simulink model "dycos10_induction_1"  (Simulink 9.2)
settings: Solver=VariableStepAuto  StartTime=0.0  StopTime=19  RelTol=1e-3
undefined symbols (not defined in the file): D1, Delta, k1, k2
libraries: powerlib x49, powerlib_meascontrol x2, factslib x1
settings Model: Creator=moham  LastModifiedBy=moham
settings DataIOCC: LimitDataPoints=off  SaveFormat=Dataset  SignalLoggingSaveFormat=Dataset  ReturnWorkspaceOutputs=on
settings OptimizationCC: LifeSpan=auto
settings DebuggingCC: UnderspecifiedInitializationDetection=Simplified  MergeDetectMultiDrivingBlocksExec=error  FcnCallInpInsideContextMsg=error  UnconnectedInputMsg=none  UnconnectedOutputMsg=none  UnconnectedLineMsg=none  StateNameClashWarn=none  SFUnexpectedBacktrackingDiag=error  SFNoUnconditionalDefaultTransitionDiag=error  SFExecutionAtInitializationDiag=warning
settings HardwareCC: ProdBitPerPointer=64  ProdBitPerSizeT=64  ProdBitPerPtrDiffT=64  ProdLargestAtomicFloat=Float  ProdIntDivRoundTo=Zero  ProdEndianess=LittleEndian  ProdWordSize=64  ProdHWDeviceType=Intel->x86-64 (Windows64)
settings ModelReferenceCC: EnableRefExpFcnMdlSchedulingChecks=off  PropagateSignalLabelsOutOfModel=on
settings SFSimCC: SimUseLocalCustomCode=on
settings RTWCC: RTWUseLocalCustomCode=on
settings CodeAppCC: StateflowObjectComments=off
settings GRTTargetCC: TargetLangStandard=C99 (ISO)  CombineOutputUpdateFcns=on  GRTInterface=off
settings ConfigComp: CovMetricSettings=dwe  CovSaveCumulativeToWorkspaceVar=off  CovSaveSingleToWorkspaceVar=off  CovExternalEMLEnable=on

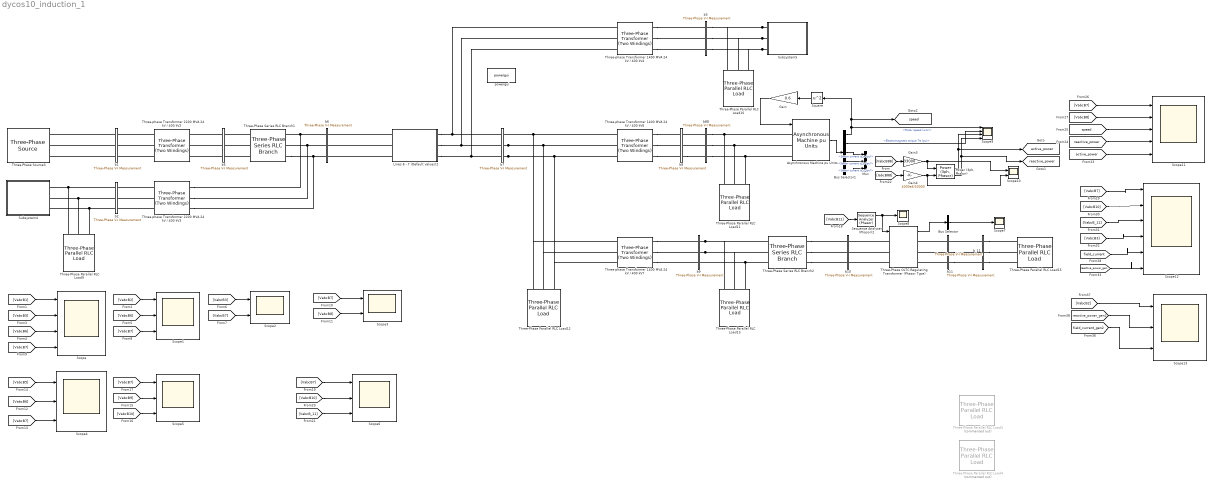
== system dycos10_induction_1 ==
  Asynchronous Machine pu Units : powerlib/Machines/Asynchronous Machine pu Units  RotorType=Squirrel-cage  PresetModel=No  MechanicalLoad=Torque Tm  ShowDetailedParameters=on  ReferenceFrame=Rotor  Units=pu  MeasurementBus=off  NominalParameters=[3600e6 33000 60]  VoltageRatio=1  Stator=[0.01 0.145]  Rotor=[0.008 0.145]  Cage1=[0.01909 0.0397]  Cage2=[0.01909 0.0397]  Lm=3.3  Mechanical=[0.6 0 2]  PolePairs=2  InitialConditions=[-6.39894e-41 0 0.310738 0.310738 0.310738 -24.5903 -144.59 95.4097]  SimulateSaturation=off  Saturation="[0.212,0.4201,0.8125,1.0979,1.4799,2.2457,3.2586,4.5763,6.4763 ;   0.5,0.7,0.9,1,1.1,1.2 ,1.3,1.4,1.5]"  LoadFlowParameters=0  TsPowergui=0  TsBlock=-1  IterativeModel=Trapezoidal non iterative  IterativeDiscreteModel=Trapezoidal non iterative  Pmec=3600e6*0.6
  Bus Selector : BusSelector  OutputSignals=Tap  OutputAsBus=on
  Bus Selector1 : BusSelector  OutputSignals=Mechanical.Rotor speed (wm),Mechanical.Electromagnetic torque Te (pu),Stator measurements.Stator current is_a (pu),Stator measurements.Stator current is_b (pu),Stator measurements.Stator current is_c (pu)
  Gain : Gain  Gain=0.6
  Gain3 : Gain  Gain=33000
  Gain4 : Gain  Gain=4000e6/33000
  Lines 6 - 7 (Default values)2 : Subsystem
  Mux : Mux  Inputs=3
  "Power (3ph, Phasor)" : powerlib_meascontrol/Measurements/Power (3ph, Phasor)
  Scope : Scope  NumInputPorts=4
  Scope{1,4..6,13} (5 alike) : Scope  NumInputPorts=3
  Scope10 : Scope  NumInputPorts=2
  Scope11 : Scope  NumInputPorts=5
  Scope12 : Scope  NumInputPorts=6
  Scope2 : Scope  NumInputPorts=2
  Scope3 : Scope  NumInputPorts=2
  Scope7 : Scope
  Scope8 : Scope
  Scope9 : Scope  NumInputPorts=4
  Sequence Analyzer (Phasor)2 : powerlib_meascontrol/Measurements/Sequence Analyzer (Phasor)  seq=Positive
  Square : Math  Operator=square  SaturateOnIntegerOverflow=on
  Subsystem4 : Subsystem
  Subsystem5 : Subsystem
  Three-Phase Parallel RLC Load10 : powerlib/Elements/Three-Phase Parallel RLC Load  LConnTagsString=A|B|C  Configuration=Y (grounded)  NominalVoltage=(24000)*1  Vabc=[1e3 1e3 1e3]  Vabcp=[1e3 1e3 1e3]  NominalFrequency=60  UnbalancedPower=off  ActivePower=5e6  InductivePower=0  CapacitivePower=0  Pabc=[10e3 9e3 11e3]  QLabc=[100 90 110]  QCabc=[100 90 110]  Pabcp=[10e3 9e3 11e3]  QLabcp=[100 90 110]  QCabcp=[100 90 110]  Measurements=None  LoadType=constant PQ
  Three-Phase Parallel RLC Load11 : powerlib/Elements/Three-Phase Parallel RLC Load  LConnTagsString=A|B|C  Configuration=Y (grounded)  NominalVoltage=(717697)*0.0445324  Vabc=[1e3 1e3 1e3]  Vabcp=[1e3 1e3 1e3]  NominalFrequency=60  UnbalancedPower=off  ActivePower=0  InductivePower=0  CapacitivePower=600*1e6  Pabc=[10e3 9e3 11e3]  QLabc=[100 90 110]  QCabc=[100 90 110]  Pabcp=[10e3 9e3 11e3]  QLabcp=[100 90 110]  QCabcp=[100 90 110]  Measurements=None  LoadType=constant PQ
  Three-Phase Parallel RLC Load12 : powerlib/Elements/Three-Phase Parallel RLC Load  LConnTagsString=A|B|C  Configuration=Y (grounded)  NominalVoltage=(8.15772e+06)*0.0445322  Vabc=[1e3 1e3 1e3]  Vabcp=[1e3 1e3 1e3]  NominalFrequency=60  UnbalancedPower=off  ActivePower=0  InductivePower=0  CapacitivePower=763*1e6  Pabc=[10e3 9e3 11e3]  QLabc=[100 90 110]  QCabc=[100 90 110]  Pabcp=[10e3 9e3 11e3]  QLabcp=[100 90 110]  QCabcp=[100 90 110]  Measurements=None  LoadType=constant PQ
  Three-Phase Parallel RLC Load13 : powerlib/Elements/Three-Phase Parallel RLC Load  LConnTagsString=A|B|C  Configuration=Y (grounded)  NominalVoltage=(726764)*0.0445322  Vabc=[1e3 1e3 1e3]  Vabcp=[1e3 1e3 1e3]  NominalFrequency=60  UnbalancedPower=off  ActivePower=0  InductivePower=0  CapacitivePower=1710*1e6  Pabc=[10e3 9e3 11e3]  QLabc=[100 90 110]  QCabc=[100 90 110]  Pabcp=[10e3 9e3 11e3]  QLabcp=[100 90 110]  QCabcp=[100 90 110]  Measurements=None  LoadType=constant PQ
  Three-Phase Parallel RLC Load15 : powerlib/Elements/Three-Phase Parallel RLC Load  LConnTagsString=A|B|C  Configuration=Y (grounded)  NominalVoltage=11e3  Vabc=[1e3 1e3 1e3]  Vabcp=[1e3 1e3 1e3]  NominalFrequency=60  UnbalancedPower=off  ActivePower=3435*1e6  InductivePower=985*1e6  CapacitivePower=0  Pabc=[10e3 9e3 11e3]  QLabc=[100 90 110]  QCabc=[100 90 110]  Pabcp=[10e3 9e3 11e3]  QLabcp=[100 90 110]  QCabcp=[100 90 110]  Measurements=None  LoadType=constant PQ
  Three-Phase Parallel RLC Load3 : powerlib/Elements/Three-Phase Parallel RLC Load  Commented=on  LConnTagsString=A|B|C  Configuration=Y (grounded)  NominalVoltage=11e3  Vabc=[1e3 1e3 1e3]  Vabcp=[1e3 1e3 1e3]  NominalFrequency=60  UnbalancedPower=off  ActivePower=k1*0.5*1e6  InductivePower=k2*0.5*1e6  CapacitivePower=0  Pabc=[10e3 9e3 11e3]  QLabc=[100 90 110]  QCabc=[100 90 110]  Pabcp=[10e3 9e3 11e3]  QLabcp=[100 90 110]  QCabcp=[100 90 110]  Measurements=None  LoadType=constant Z
  Three-Phase Parallel RLC Load4 : powerlib/Elements/Three-Phase Parallel RLC Load  Commented=on  LConnTagsString=A|B|C  Configuration=Y (grounded)  NominalVoltage=11e3  Vabc=[1e3 1e3 1e3]  Vabcp=[1e3 1e3 1e3]  NominalFrequency=60  UnbalancedPower=off  ActivePower=k1*0.5*1e6  InductivePower=k2*0.5*1e6  CapacitivePower=0  Pabc=[10e3 9e3 11e3]  QLabc=[100 90 110]  QCabc=[100 90 110]  Pabcp=[10e3 9e3 11e3]  QLabcp=[100 90 110]  QCabcp=[100 90 110]  Measurements=None  LoadType=constant I
  Three-Phase Parallel RLC Load9 : powerlib/Elements/Three-Phase Parallel RLC Load  LConnTagsString=A|B|C  Configuration=Y (grounded)  NominalVoltage=(24000)*1  Vabc=[1e3 1e3 1e3]  Vabcp=[1e3 1e3 1e3]  NominalFrequency=60  UnbalancedPower=off  ActivePower=5e6  InductivePower=0  CapacitivePower=0  Pabc=[10e3 9e3 11e3]  QLabc=[100 90 110]  QCabc=[100 90 110]  Pabcp=[10e3 9e3 11e3]  QLabcp=[100 90 110]  QCabcp=[100 90 110]  Measurements=None  LoadType=constant PQ
  Three-Phase Series RLC Branch1 : powerlib/Elements/Three-Phase Series RLC Branch  LConnTagsString=A|B|C  RConnTagsString=A|B|C  BranchType=L  Resistance=1  Inductance=1e-3  Capacitance=1e-6  Measurements=None
  Three-Phase Series RLC Branch2 : powerlib/Elements/Three-Phase Series RLC Branch  LConnTagsString=A|B|C  RConnTagsString=A|B|C  BranchType=RL  Resistance=0.005  Inductance=0.08e-3  Capacitance=1e-6  Measurements=None
  Three-Phase OLTC Regulating Transformer (Phasor Type) : factslib/Transformers/Three-Phase OLTC Regulating Transformer (Phasor Type)  Winding1Connection=Yg  Winding2Connection=Yg  PnomFnom="[4000e6,  60]"  Winding1=[33e3, 0 , 0.001*40 ]  Winding2="[11e3,  0, 0.001*40 ]"  Iw2_init=[0.75/528, -45]  RmXm=[500, 500]  TapOnWinding=Winding 2  WindingTap=[ 0, 0.0001*40]  dU=0.00625  TapMinMax=[ -16, +16]  InitialTap=0  TapSelectionTime=1.5  ExternalControl=off  RegulatorOn=on  Regulator="[.84,  0.01, 0]"
      link override Rm_Xm_1: ActivePower=4000000  InductivePower=4000000
      link override Rm_Xm_2: ActivePower=4000000  InductivePower=4000000
  Three-Phase Source3 : powerlib/Electrical Sources/Three-Phase Source  InternalConnection=Yg  VoltagePhases=off  Voltage=(24000)*1  PhaseAngle=0  Voltage_phases=[25e3 25e3 25e3]/sqrt(3)  PhaseAngles_phases=[0 -120 +120]  Frequency=60  NonIdealSource=off  SpecifyImpedance=off  Resistance=0.8929  Inductance=16.58e-3  ShortCircuitLevel=100e6  BaseVoltage=24e3  XRratio=7  BusType=swing  Pref=50000000000  Qref=0  Prefabc=[10e3, 10e3, 10e3]  Qrefabc=[0, 0, 0]  Qmin=-Inf  Qmax=Inf
  Three-phase Transformer 1400 MVA 24 kV / 400 kV4 : powerlib/Elements/Three-Phase Transformer (Two Windings)  Winding1Connection=Delta (D1)  Winding2Connection=Yg  CoreType=Three single-phase transformers  SetSaturation=off  Hysteresis=off  DataFile='hysteresis'  SetInitialFlux=off  Measurements=None  UNITS=pu  NominalPower=[ 1400e6 60 ]  Winding1="[ 24e3 0  0.0125*14]"  Winding2=[ 400e3*0.9024 0 0.0125*14/(17*17)]  Rm=500  Lm=500  L0=0.5  Saturation="[ 0,0  ;  0.005,1.2  ;  1.0,1.4 ]"  InitialFluxes=[ 0.8 , -0.8 , 0.7 ]  BreakLoop=off  DiscreteSolver=Trapezoidal iterative  DataType=off  TransfoNumber=0
  Three-phase Transformer 1400 MVA 24 kV / 400 kV6 : powerlib/Elements/Three-Phase Transformer (Two Windings)  Winding1Connection=Delta (D1)  Winding2Connection=Yg  CoreType=Three single-phase transformers  SetSaturation=off  Hysteresis=off  DataFile='hysteresis'  SetInitialFlux=off  Measurements=None  UNITS=pu  NominalPower=[ 4000e6 60 ]  Winding1="[ 400e3 0  0.003*40/(12*12)]"  Winding2=[ 33e3*1.0664 0 0.003*40]  Rm=500  Lm=500  L0=0.5  Saturation="[ 0,0  ;  0.005,1.2  ;  1.0,1.4 ]"  InitialFluxes=[ 0.8 , -0.8 , 0.7 ]  BreakLoop=off  DiscreteSolver=Trapezoidal iterative  DataType=off  TransfoNumber=0
  Three-phase Transformer 1400 MVA 24 kV / 400 kV7 : powerlib/Elements/Three-Phase Transformer (Two Windings)  Winding1Connection=Delta (D1)  Winding2Connection=Yg  CoreType=Three single-phase transformers  SetSaturation=off  Hysteresis=off  DataFile='hysteresis'  SetInitialFlux=off  Measurements=None  UNITS=pu  NominalPower=[ 4000e6 60 ]  Winding1="[ 400e3 0  0.0026*40/144]"  Winding2=[ 33e3*1.08 0 0.0026*40]  Rm=500  Lm=500  L0=0.5  Saturation="[ 0,0  ;  0.005,1.2  ;  1.0,1.4 ]"  InitialFluxes=[ 0.8 , -0.8 , 0.7 ]  BreakLoop=off  DiscreteSolver=Trapezoidal iterative  DataType=off  TransfoNumber=0
  Three-phase Transformer 2200 MVA 24 kV / 400 kV2 : powerlib/Elements/Three-Phase Transformer (Two Windings)  Winding1Connection=Delta (D1)  Winding2Connection=Yg  CoreType=Three single-phase transformers  SetSaturation=off  Hysteresis=off  DataFile='hysteresis'  SetInitialFlux=off  Measurements=None  UNITS=pu  NominalPower=[ 4000e6 60 ]  Winding1="[ 24e3 0  0.002/400]"  Winding2=[ 400e3*0.8857 0 0.002/400]  Rm=1000  Lm=1000  L0=0.5  Saturation="[ 0,0  ;  0.005,1.2  ;  1.0,1.4 ]"  InitialFluxes=[ 0.8 , -0.8 , 0.7 ]  BreakLoop=off  DiscreteSolver=Trapezoidal iterative  DataType=off  TransfoNumber=0
  Three-phase Transformer 2200 MVA 24 kV / 400 kV3 : powerlib/Elements/Three-Phase Transformer (Two Windings)  Winding1Connection=Delta (D1)  Winding2Connection=Yg  CoreType=Three single-phase transformers  SetSaturation=off  Hysteresis=off  DataFile='hysteresis'  SetInitialFlux=off  Measurements=None  UNITS=pu  NominalPower=[ 2200e6 60 ]  Winding1="[ 24e3 0  0.0045*22]"  Winding2=[ 400e3*0.8857 0 0.0045*22/(17*17)]  Rm=500  Lm=500  L0=0.5  Saturation="[ 0,0  ;  0.005,1.2  ;  1.0,1.4 ]"  InitialFluxes=[ 0.8 , -0.8 , 0.7 ]  BreakLoop=off  DiscreteSolver=Trapezoidal iterative  DataType=off  TransfoNumber=0
  b1 : powerlib/Measurements/Three-Phase V-I Measurement  VoltageMeasurement=phase-to-ground  SetLabelV=on  LabelV=VabcB1  Vpu=on  VpuLL=off  CurrentMeasurement=yes  SetLabelI=on  LabelI=IabcB1  Ipu=on  Pbase=4000e6  Vbase=24e3  OutputType=Magnitude  PhasorSimulation=on  PSBequivalent=0
  b10 : powerlib/Measurements/Three-Phase V-I Measurement  VoltageMeasurement=phase-to-ground  SetLabelV=on  LabelV=VabcB10  Vpu=on  VpuLL=off  CurrentMeasurement=yes  SetLabelI=on  LabelI=IabcB10  Ipu=on  Pbase=4000e6  Vbase=33e3  OutputType=Magnitude  PhasorSimulation=on  PSBequivalent=0
  b11 : powerlib/Measurements/Three-Phase V-I Measurement  VoltageMeasurement=phase-to-ground  SetLabelV=on  LabelV=VabcB11  Vpu=on  VpuLL=off  CurrentMeasurement=yes  SetLabelI=on  LabelI=IabcB11  Ipu=on  Pbase=4000e6  Vbase=11e3  OutputType=Complex  PhasorSimulation=on  PSBequivalent=0
  b2 : powerlib/Measurements/Three-Phase V-I Measurement  VoltageMeasurement=phase-to-ground  SetLabelV=on  LabelV=VabcB2  Vpu=on  VpuLL=off  CurrentMeasurement=yes  SetLabelI=on  LabelI=IabcB2  Ipu=on  Pbase=2200e6  Vbase=24e3  OutputType=Magnitude  PhasorSimulation=on  PSBequivalent=0
  b3 : powerlib/Measurements/Three-Phase V-I Measurement  VoltageMeasurement=phase-to-phase  SetLabelV=on  LabelV=VabcB3  Vpu=on  VpuLL=off  CurrentMeasurement=yes  SetLabelI=on  LabelI=IabcB3  Ipu=on  Pbase=1100e6  Vbase=24e3  OutputType=Magnitude  PhasorSimulation=on  PSBequivalent=0
  b5 : powerlib/Measurements/Three-Phase V-I Measurement  VoltageMeasurement=phase-to-ground  SetLabelV=on  LabelV=VabcB5  Vpu=on  VpuLL=off  CurrentMeasurement=yes  SetLabelI=on  LabelI=IabcB5  Ipu=on  Pbase=4000e6  Vbase=400e3  OutputType=Magnitude  PhasorSimulation=on  PSBequivalent=0
  b6 : powerlib/Measurements/Three-Phase V-I Measurement  VoltageMeasurement=phase-to-ground  SetLabelV=on  LabelV=VabcB6  Vpu=on  VpuLL=off  CurrentMeasurement=yes  SetLabelI=on  LabelI=IabcB6  Ipu=on  Pbase=4000e6  Vbase=400e3  OutputType=Magnitude  PhasorSimulation=on  PSBequivalent=0
  b7 : powerlib/Measurements/Three-Phase V-I Measurement  VoltageMeasurement=phase-to-ground  SetLabelV=on  LabelV=VabcB7  Vpu=on  VpuLL=off  CurrentMeasurement=yes  SetLabelI=on  LabelI=IabcB7  Ipu=on  Pbase=4000e6  Vbase=400e3  OutputType=Magnitude  PhasorSimulation=on  PSBequivalent=0
  b8 : powerlib/Measurements/Three-Phase V-I Measurement  VoltageMeasurement=phase-to-ground  SetLabelV=on  LabelV=VabcB8  Vpu=on  VpuLL=off  CurrentMeasurement=yes  SetLabelI=on  LabelI=IabcB8  Ipu=on  Pbase=4000e6  Vbase=33e3  OutputType=Magnitude  PhasorSimulation=on  PSBequivalent=0
  b88 : powerlib/Measurements/Three-Phase V-I Measurement  VoltageMeasurement=phase-to-ground  SetLabelV=on  LabelV=VabcB88  Vpu=on  VpuLL=off  CurrentMeasurement=yes  SetLabelI=on  LabelI=IabcB88  Ipu=on  Pbase=4000e6  Vbase=33e3  OutputType=Complex  PhasorSimulation=on  PSBequivalent=0
  b9 : powerlib/Measurements/Three-Phase V-I Measurement  VoltageMeasurement=phase-to-ground  SetLabelV=on  LabelV=VabcB9  Vpu=on  VpuLL=off  CurrentMeasurement=yes  SetLabelI=on  LabelI=IabcB9  Ipu=on  Pbase=4000e6  Vbase=33e3  OutputType=Magnitude  PhasorSimulation=on  PSBequivalent=0
  b_11 : powerlib/Measurements/Three-Phase V-I Measurement  VoltageMeasurement=phase-to-ground  SetLabelV=on  LabelV=VabcB_11  Vpu=on  VpuLL=off  CurrentMeasurement=yes  SetLabelI=on  LabelI=IabcB_11  Ipu=on  Pbase=4000e6  Vbase=11e3  OutputType=Magnitude  PhasorSimulation=on  PSBequivalent=0
  powergui : powerlib/powergui  Priority=1  SimulationMode=Phasor  SampleTime=5e-6  frequency=60  Iterations=50  frequencyindice=60  Pbase=100e6  ErrMax=1e-4  UnitsV=kV  UnitsW=MW  buscounter=0  FunctionMessages=off  echomessages=off  EnableUseOfTLC=off  CurrentSourceSwitches=off  DisableSnubberDevices=off  DisableRonSwitches=off  DisableVfSwitches=off  DisplayEquations=off  AutomaticDiscreteSolvers=off  SolverType=Tustin/Backward Euler (TBE)  Interpol=off  ExternalGateDelay=off  methode=off  Ts=100  x0status=blocks  SPID=on  SwTol=0  HookPort=off  NonlinearTolerance=1e-4  nMaxIteration=100  ContinueOnMaxIteration=off  RestoreLinks=warning  ResistiveCurrentMeasurement=off  Frange=[0:2:500]  Ylog=off  Xlog=on  ShowGrid=off  save=off  variable=ZData  structure=0  ZoomFFT=off  StartTime=0.0  cycles=1  DisplayStyle=1  fundamental=60  FreqAxis=off  MaxFrequency=1000  frequencyindicesteady=1  RmsSteady=1  display=off
  tag scope: active_power=global, reactive_power=global, speed=global
  wires:
  [VabcB7] -> Scope6/1
  [VabcB10] -> Scope6/2
  [VabcB7] -> Scope/4
  Bus Selector/1 -> Scope7/1
  Sequence Analyzer (Phasor)2/1 -> Scope8/1, Three-Phase OLTC Regulating Transformer (Phasor Type)/1
  [VabcB7] -> Scope5/1
  [VabcB11] -> Sequence Analyzer (Phasor)2/1
  [VabcB7] -> Scope2/2
  [VabcB2] -> Scope1/1
  [VabcB10] -> Scope5/3
  [VabcB3] -> Scope2/1
  [VabcB5] -> Scope4/1
  [VabcB9] -> Scope5/2
  [VabcB5] -> Scope/2
  [VabcB7] -> Scope4/3
  Three-Phase OLTC Regulating Transformer (Phasor Type)/1 -> Bus Selector/1
  [VabcB6] -> Scope4/2
  [VabcB7] -> Scope3/1
  [VabcB7] -> Scope1/3
  [VabcB_11] -> Scope6/3
  [VabcB1] -> Scope/1
  [VabcB6] -> Scope1/2
  [VabcB8] -> Scope3/2
  [VabcB6] -> Scope/3
  Asynchronous Machine pu Units/1 -> Bus Selector1/1
  Bus Selector1/1 -> [speed], Square/1, Scope9/1  "<Rotor speed (wm)>"
  Square/1 -> Gain/1
  Gain/1 -> Asynchronous Machine pu Units/1
  Bus Selector1/2 -> Scope9/2  "<Electromagnetic torque Te (pu)>"
  Bus Selector1/3 -> Mux/1  "<Stator current is_a (pu)>"
  Bus Selector1/4 -> Mux/2  "<Stator current is_b (pu)>"
  Bus Selector1/5 -> Mux/3  "<Stator current is_c (pu)>"
  "Power (3ph, Phasor)"/1 -> [active_power], Scope9/3
  "Power (3ph, Phasor)"/2 -> [reactive_power], Scope9/4
  Gain4/1 -> "Power (3ph, Phasor)"/2, Scope10/2
  Gain3/1 -> "Power (3ph, Phasor)"/1, Scope10/1
  [VabcB88] -> Gain3/1
  [IabcB88] -> Gain4/1
  [VabcB7] -> Scope11/1
  [VabcB8] -> Scope11/2
  [speed] -> Scope11/3
  [reactive_power] -> Scope11/4
  [active_power] -> Scope11/5
  [VabcB_11] -> Scope12/3
  [field_current] -> Scope12/5
  [VabcB10] -> Scope12/2
  [VabcB7] -> Scope12/1
  [VabcB3] -> Scope12/4
  [reactive_power_gen] -> Scope12/6
  [field_current_gen2] -> Scope13/3
  [reactive_power_gen2] -> Scope13/2
  [VabcB2] -> Scope13/1
  connections:
  Three-phase Transformer 1400 MVA 24 kV / 400 kV6/LConn1 -- Three-Phase Parallel RLC Load12/LConn1 -- Three-phase Transformer 1400 MVA 24 kV / 400 kV7/LConn1 -- b7/RConn1
  Three-phase Transformer 2200 MVA 24 kV / 400 kV3/RConn1 -- b6/LConn1 -- Three-Phase Series RLC Branch1/RConn1
  Subsystem5/RConn2 -- Three-Phase Parallel RLC Load10/LConn2 -- b3/LConn2
  Three-Phase Parallel RLC Load13/LConn3 -- b9/RConn3 -- Three-Phase Series RLC Branch2/LConn3
  Three-phase Transformer 2200 MVA 24 kV / 400 kV3/RConn2 -- b6/LConn2 -- Three-Phase Series RLC Branch1/RConn2
  b7/RConn2 -- Three-Phase Parallel RLC Load12/LConn2 -- Three-phase Transformer 1400 MVA 24 kV / 400 kV7/LConn2 -- Three-phase Transformer 1400 MVA 24 kV / 400 kV6/LConn2
  Lines 6 - 7 (Default values)2/RConn2 -- Three-phase Transformer 1400 MVA 24 kV / 400 kV4/RConn2 -- b7/LConn2
  Three-Phase Series RLC Branch1/RConn3 -- Three-phase Transformer 2200 MVA 24 kV / 400 kV3/RConn3 -- b6/LConn3
  b7/RConn3 -- Three-Phase Parallel RLC Load12/LConn3 -- Three-phase Transformer 1400 MVA 24 kV / 400 kV7/LConn3 -- Three-phase Transformer 1400 MVA 24 kV / 400 kV6/LConn3
  b9/RConn1 -- Three-Phase Parallel RLC Load13/LConn1 -- Three-Phase Series RLC Branch2/LConn1
  Three-Phase Parallel RLC Load9/LConn3 -- b2/LConn3 -- Subsystem4/RConn3
  Three-Phase Parallel RLC Load9/LConn1 -- b2/LConn1 -- Subsystem4/RConn1
  Lines 6 - 7 (Default values)2/RConn1 -- Three-phase Transformer 1400 MVA 24 kV / 400 kV4/RConn1 -- b7/LConn1
  Subsystem5/RConn3 -- b3/LConn3 -- Three-Phase Parallel RLC Load10/LConn3
  Subsystem5/RConn1 -- Three-Phase Parallel RLC Load10/LConn1 -- b3/LConn1
  Three-Phase Parallel RLC Load9/LConn2 -- b2/LConn2 -- Subsystem4/RConn2
  b88/LConn2 -- b8/RConn2
  b88/LConn1 -- b8/RConn1
  Lines 6 - 7 (Default values)2/RConn3 -- Three-phase Transformer 1400 MVA 24 kV / 400 kV4/RConn3 -- b7/LConn3
  b9/RConn2 -- Three-Phase Parallel RLC Load13/LConn2 -- Three-Phase Series RLC Branch2/LConn2
  Three-Phase Parallel RLC Load11/LConn3 -- Asynchronous Machine pu Units/LConn3 -- b88/RConn3
  Three-phase Transformer 1400 MVA 24 kV / 400 kV4/LConn1 -- b3/RConn1
  b11/RConn3 -- b_11/LConn3
  Three-phase Transformer 2200 MVA 24 kV / 400 kV2/LConn3 -- b1/RConn3
  b_11/RConn1 -- Three-Phase Parallel RLC Load15/LConn1
  b_11/RConn3 -- Three-Phase Parallel RLC Load15/LConn3
  Three-Phase Series RLC Branch2/RConn3 -- b10/LConn3
  b5/LConn3 -- Three-phase Transformer 2200 MVA 24 kV / 400 kV2/RConn3
  Three-Phase OLTC Regulating Transformer (Phasor Type)/LConn3 -- b10/RConn3
  Three-phase Transformer 1400 MVA 24 kV / 400 kV7/RConn2 -- b9/LConn2
  Three-Phase OLTC Regulating Transformer (Phasor Type)/LConn2 -- b10/RConn2
  Three-phase Transformer 1400 MVA 24 kV / 400 kV6/RConn3 -- b8/LConn3
  Three-Phase Series RLC Branch1/LConn2 -- b5/RConn2
  Three-Phase Series RLC Branch2/RConn2 -- b10/LConn2
  Three-phase Transformer 1400 MVA 24 kV / 400 kV4/LConn3 -- b3/RConn3
  Three-phase Transformer 1400 MVA 24 kV / 400 kV4/LConn2 -- b3/RConn2
  Three-Phase Series RLC Branch1/LConn1 -- b5/RConn1
  b5/LConn1 -- Three-phase Transformer 2200 MVA 24 kV / 400 kV2/RConn1
  Lines 6 - 7 (Default values)2/LConn2 -- b6/RConn2
  b_11/LConn1 -- b11/RConn1
  Three-phase Transformer 2200 MVA 24 kV / 400 kV3/LConn1 -- b2/RConn1
  Three-Phase Series RLC Branch2/RConn1 -- b10/LConn1
  Three-phase Transformer 2200 MVA 24 kV / 400 kV2/LConn1 -- b1/RConn1
  b1/LConn1 -- Three-Phase Source3/RConn1
  Lines 6 - 7 (Default values)2/LConn3 -- b6/RConn3
  b11/LConn2 -- Three-Phase OLTC Regulating Transformer (Phasor Type)/RConn2
  b11/LConn3 -- Three-Phase OLTC Regulating Transformer (Phasor Type)/RConn3
  Three-phase Transformer 1400 MVA 24 kV / 400 kV6/RConn1 -- b8/LConn1
  Three-Phase OLTC Regulating Transformer (Phasor Type)/LConn1 -- b10/RConn1
  b_11/RConn2 -- Three-Phase Parallel RLC Load15/LConn2
  Three-Phase Series RLC Branch1/LConn3 -- b5/RConn3
  b1/LConn2 -- Three-Phase Source3/RConn2
  Three-phase Transformer 2200 MVA 24 kV / 400 kV3/LConn2 -- b2/RConn2
  Three-phase Transformer 1400 MVA 24 kV / 400 kV6/RConn2 -- b8/LConn2
  Three-phase Transformer 2200 MVA 24 kV / 400 kV2/LConn2 -- b1/RConn2
  Three-phase Transformer 1400 MVA 24 kV / 400 kV7/RConn1 -- b9/LConn1
  b11/RConn2 -- b_11/LConn2
  b11/LConn1 -- Three-Phase OLTC Regulating Transformer (Phasor Type)/RConn1
  b1/LConn3 -- Three-Phase Source3/RConn3
  Three-phase Transformer 2200 MVA 24 kV / 400 kV3/LConn3 -- b2/RConn3
  Lines 6 - 7 (Default values)2/LConn1 -- b6/RConn1
  Three-phase Transformer 1400 MVA 24 kV / 400 kV7/RConn3 -- b9/LConn3
  b5/LConn2 -- Three-phase Transformer 2200 MVA 24 kV / 400 kV2/RConn2
  Three-Phase Parallel RLC Load11/LConn1 -- Asynchronous Machine pu Units/LConn1 -- b88/RConn1
  Three-Phase Parallel RLC Load11/LConn2 -- b88/RConn2 -- Asynchronous Machine pu Units/LConn2
  b8/RConn3 -- b88/LConn3

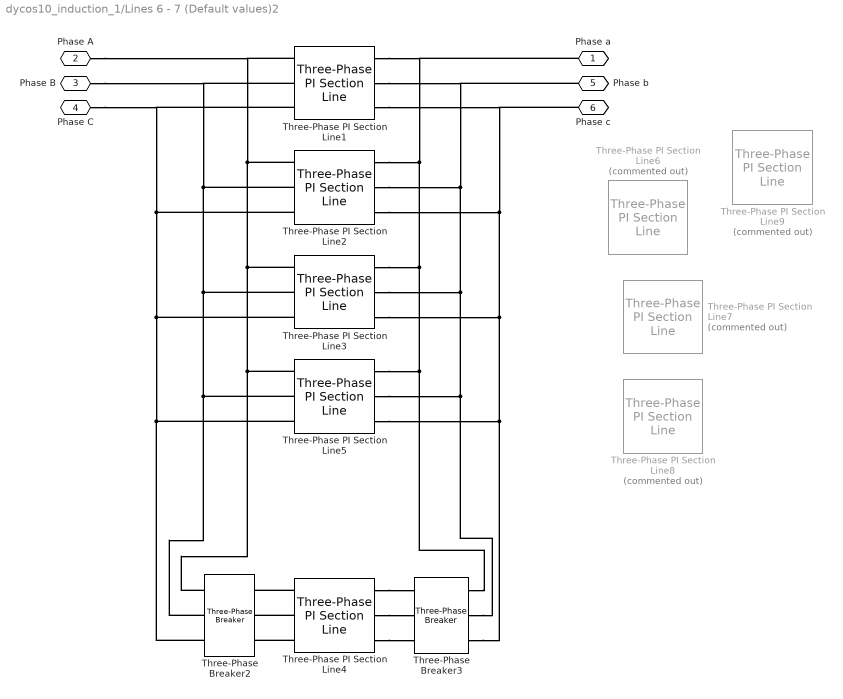
== system dycos10_induction_1/Lines 6 - 7 (Default values)2 ==
  Three-Phase PI Section Line{1..5} (5 alike) : powerlib/Elements/Three-Phase PI Section Line  LConnTagsString=a|b|c  RConnTagsString=A|B|C  Length=10  Frequency=60  Resistances=[ 0.15 3*0.15] *10 /10  Inductances="[15e-3  3*0.0072]*10 /10"  Capacitances=[23.4e-6 70e-6]/(50*2)
  Three-Phase PI Section Line6 : powerlib/Elements/Three-Phase PI Section Line  Commented=on  LConnTagsString=a|b|c  RConnTagsString=A|B|C  Length=10  Frequency=60  Resistances=[ 1e-6*3.75*5/10 3*1e-6*3.75*5/10]  Inductances="[5*1e-6*7.2/10  3*5*1e-6*7.2/10]"  Capacitances=[300*1e-6/50 3*300*1e-6/50]
  Three-Phase PI Section Line7 : powerlib/Elements/Three-Phase PI Section Line  Commented=on  LConnTagsString=a|b|c  RConnTagsString=A|B|C  Length=10  Frequency=60  Resistances=[ 2e-3*0.4*5*120*pi/10 3*2e-3*0.4*5*120*pi/10]  Inductances="[5*2e-3*7.2/10  3*5*2e-3*7.2/10]"  Capacitances=[300*2e-3/50 3*300*2e-3/50]
  Three-Phase PI Section Line8 : powerlib/Elements/Three-Phase PI Section Line  Commented=on  LConnTagsString=a|b|c  RConnTagsString=A|B|C  Length=10  Frequency=60  Resistances=[ 0.15 3*0.15] *5 /10  Inductances="[7.2e-3  3*0.0072]*5 /10"  Capacitances=[23.4e-6 70e-6]/50
  Three-Phase PI Section Line9 : powerlib/Elements/Three-Phase PI Section Line  Commented=on  LConnTagsString=a|b|c  RConnTagsString=A|B|C  Length=10  Frequency=60  Resistances=[ 0.15 3*0.15] *10 /10  Inductances="[7.2e-3  3*0.0072]*10 /10"  Capacitances=[23.4e-6 70e-6]/(50*2)
  Three-Phase Breaker2 : powerlib/Elements/Three-Phase Breaker  InitialState=closed  SwitchA=on  SwitchB=on  SwitchC=on  SwitchTimes="[100  300]"  External=off  BreakerResistance=0.01  SnubberResistance=1e6  SnubberCapacitance=inf  Measurements=None
  Three-Phase Breaker3 : powerlib/Elements/Three-Phase Breaker  InitialState=closed  SwitchA=on  SwitchB=on  SwitchC=on  SwitchTimes="[100  300]"  External=off  BreakerResistance=0.01  SnubberResistance=1e6  SnubberCapacitance=inf  Measurements=None
  Phase a : PMIOPort  Side=Right
  Phase A : PMIOPort  Port=2  Side=Left
  Phase B : PMIOPort  Port=3  Side=Left
  Phase C : PMIOPort  Port=4  Side=Left
  Phase b : PMIOPort  Port=5  Side=Right
  Phase c : PMIOPort  Port=6  Side=Right
  connections:
  Three-Phase Breaker2/LConn1 -- Three-Phase PI Section Line5/LConn1 -- Three-Phase PI Section Line3/LConn1 -- Three-Phase PI Section Line2/LConn1 -- Three-Phase PI Section Line1/LConn1 -- Phase A/RConn1
  Three-Phase Breaker2/LConn2 -- Three-Phase PI Section Line5/LConn2 -- Three-Phase PI Section Line3/LConn2 -- Three-Phase PI Section Line2/LConn2 -- Three-Phase PI Section Line1/LConn2 -- Phase B/RConn1
  Three-Phase Breaker2/LConn3 -- Three-Phase PI Section Line5/LConn3 -- Three-Phase PI Section Line3/LConn3 -- Three-Phase PI Section Line2/LConn3 -- Three-Phase PI Section Line1/LConn3 -- Phase C/RConn1
  Three-Phase Breaker3/RConn1 -- Three-Phase PI Section Line5/RConn1 -- Three-Phase PI Section Line3/RConn1 -- Three-Phase PI Section Line2/RConn1 -- Three-Phase PI Section Line1/RConn1 -- Phase a/RConn1
  Three-Phase Breaker3/RConn2 -- Three-Phase PI Section Line5/RConn2 -- Three-Phase PI Section Line3/RConn2 -- Three-Phase PI Section Line2/RConn2 -- Three-Phase PI Section Line1/RConn2 -- Phase b/RConn1
  Three-Phase Breaker3/RConn3 -- Three-Phase PI Section Line5/RConn3 -- Three-Phase PI Section Line3/RConn3 -- Three-Phase PI Section Line2/RConn3 -- Three-Phase PI Section Line1/RConn3 -- Phase c/RConn1
  Three-Phase PI Section Line4/RConn2 -- Three-Phase Breaker3/LConn2
  Three-Phase PI Section Line4/RConn3 -- Three-Phase Breaker3/LConn3
  Three-Phase PI Section Line4/LConn3 -- Three-Phase Breaker2/RConn3
  Three-Phase PI Section Line4/RConn1 -- Three-Phase Breaker3/LConn1
  Three-Phase PI Section Line4/LConn1 -- Three-Phase Breaker2/RConn1
  Three-Phase PI Section Line4/LConn2 -- Three-Phase Breaker2/RConn2

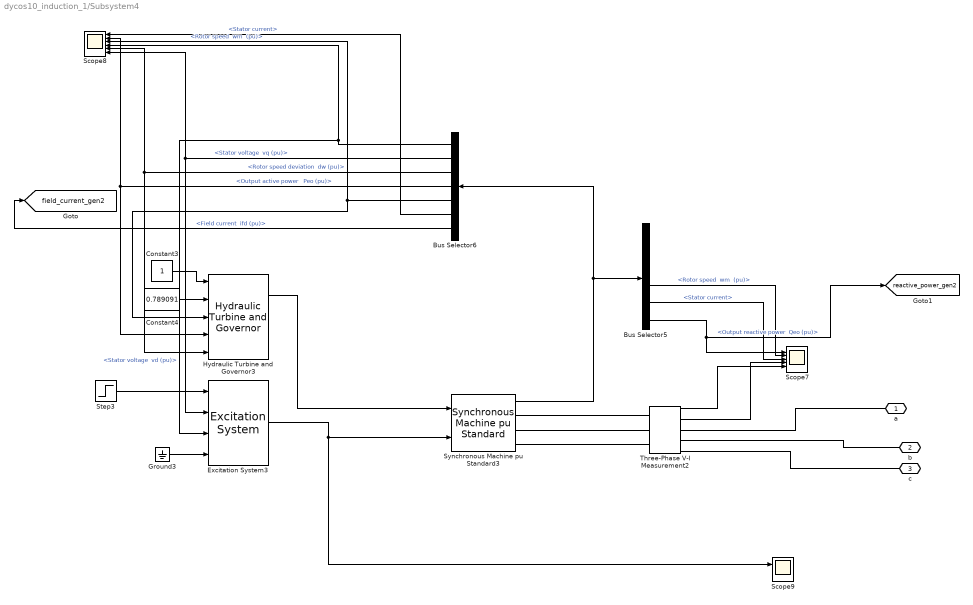
== system dycos10_induction_1/Subsystem4 ==
  Bus Selector5 : BusSelector  OutputSignals="dq0 components.Stator voltage  vd (pu),dq0 components.Stator voltage  vq (pu),Output active power   Peo (pu),Mechanical.Rotor speed  wm  (pu),Stator current,Output reactive power  Qeo (pu)"
  Bus Selector6 : BusSelector  OutputSignals="dq0 components.Stator voltage  vd (pu),dq0 components.Stator voltage  vq (pu),Mechanical.Rotor speed deviation  dw (pu),Output active power   Peo (pu),Mechanical.Rotor speed  wm  (pu),Stator current,dq0 components.Field current  ifd (pu)"
  Constant3 : Constant
  Constant4 : Constant  Value=0.789091
  Excitation System3 : powerlib/Machines/Excitation System  tr=20e-3  reg=[ 300, 0.001 ]  exc=[ 1, 0 ]  tgr=[ 0, 0 ]  damp=[ 0.001, 0.1 ]  sat=[ 0, 0 ]  lim=[ -11.5, 11.5, 0 ]  v0=[1,1.89699]
  Ground3 : Ground
  Hydraulic Turbine and Governor3 : powerlib/Machines/Hydraulic Turbine and Governor  sm="[ 10/3  0.07 ]"  gate="[  0.01  0.97518  -0.1  0.1 ]"  reg="[  0.05  1.163  0.105  0  0.01  ]"  hyd="[  0  2.67  ]"  dref=0  po=0.791957
  Scope7 : Scope  NumInputPorts=5
  Scope8 : Scope  NumInputPorts=6
  Scope9 : Scope  NumInputPorts=2
  Step3 : Step  Time=0  Before=1  SampleTime=0
  Synchronous Machine pu Standard3 : powerlib/Machines/Synchronous Machine pu Standard  PresetModel=No  MechanicalLoad=Mechanical power Pm  ShowDetailedParameters=on  RotorType=Salient-pole  Units=per unit standard parameters  MeasurementBus=off  NominalParameters=[2200e+06 24000 60]  Reactances1=[ 1.81, 0.3, 0.23, 1.76, 0.65, 0.25, 0.15 ]  Reactances2=[2.07 0.28 0.215 1.99 0.215 0.155]  dAxisTimeConstants=Open-circuit  qAxisTimeConstants=Open-circuit  TimeConstants1="[ 4.1  0.033  0.062  ]"  TimeConstants2=[ 8.0, 0.03, 1.0, 0.07 ]  TimeConstants3="[  4.49  0.0681  0.0513  ]"  TimeConstants4=[ 8.0, 0.03, 0.3371, 0.0295 ]  TimeConstants5=[ 1.01, 0.053, 0.1 ]  TimeConstants6=[ 1.3201, 0.023, 1.0, 0.07 ]  TimeConstants7=[4.1 0.033 0.062]  TimeConstants8=[ 1.3201, 0.0231, 0.3371, 0.0295 ]  StatorResistance=0.0046  Mechanical=[2.09 0 2]  PolePairs=20  InitialConditions=[0 -26.6647 0.789311 0.789311 0.789311 6.29959 -113.7 126.3 1.89699]  SetSaturation=off  Saturation=[0.6404,0.7127,0.8441,0.9214,0.9956,1.082,1.19,1.316,1.457;0.7,0.7698,0.8872,0.9466,0.9969,1.046,1.1,1.151,1.201]  LoadFlowParameters=[1 1736000000 0 0 0]  TsPowergui=0  TsBlock=-1  IterativeModel=Trapezoidal non iterative  IterativeDiscreteModel=Trapezoidal non iterative  BusType=PV  Pref=1736000000  Qref=0  Qmin=-Inf  Qmax=Inf  PLF=0  QLF=0
  Three-Phase V-I Measurement2 : powerlib/Measurements/Three-Phase V-I Measurement  VoltageMeasurement=phase-to-ground  SetLabelV=off  LabelV=Vabc  Vpu=on  VpuLL=off  CurrentMeasurement=yes  SetLabelI=off  LabelI=Iabc  Ipu=on  Pbase=2200e6  Vbase=24e3  OutputType=Magnitude  PhasorSimulation=on  PSBequivalent=0
  a : PMIOPort  Side=Right
  b : PMIOPort  Port=2  Side=Right
  c : PMIOPort  Port=3  Side=Right
  tag scope: field_current_gen2=global, reactive_power_gen2=global
  wires:
  Three-Phase V-I Measurement2/1 -> Scope7/5
  Bus Selector6/1 -> Scope8/4, Excitation System3/3  "<Stator voltage  vd (pu)>"
  Bus Selector6/2 -> Scope8/6, Excitation System3/2  "<Stator voltage  vq (pu)>"
  Synchronous Machine pu Standard3/1 -> Bus Selector5/1, Bus Selector6/1
  Hydraulic Turbine and Governor3/1 -> Synchronous Machine pu Standard3/1
  Three-Phase V-I Measurement2/2 -> Scope7/4
  Bus Selector5/5 -> Scope7/3  "<Stator current>"
  Bus Selector6/4 -> Hydraulic Turbine and Governor3/4, Scope8/2  "<Output active power   Peo (pu)>"
  Step3/1 -> Excitation System3/1
  Ground3/1 -> Excitation System3/4
  Excitation System3/1 -> Synchronous Machine pu Standard3/2, Scope9/1
  Bus Selector6/3 -> Hydraulic Turbine and Governor3/5, Scope8/5  "<Rotor speed deviation  dw (pu)>"
  Bus Selector6/5 -> Hydraulic Turbine and Governor3/3, Scope8/3  "<Rotor speed  wm  (pu)>"
  Constant3/1 -> Hydraulic Turbine and Governor3/1
  Bus Selector5/4 -> Scope7/2  "<Rotor speed  wm  (pu)>"
  Constant4/1 -> Hydraulic Turbine and Governor3/2
  Bus Selector6/6 -> Scope8/1  "<Stator current>"
  Bus Selector5/6 -> [reactive_power_gen2], Scope7/1  "<Output reactive power  Qeo (pu)>"
  Bus Selector6/7 -> [field_current_gen2]  "<Field current  ifd (pu)>"
  connections:
  Three-Phase V-I Measurement2/RConn3 -- c/RConn1
  a/RConn1 -- Three-Phase V-I Measurement2/RConn1
  Three-Phase V-I Measurement2/LConn2 -- Synchronous Machine pu Standard3/RConn2
  Three-Phase V-I Measurement2/LConn1 -- Synchronous Machine pu Standard3/RConn1
  Three-Phase V-I Measurement2/LConn3 -- Synchronous Machine pu Standard3/RConn3
  b/RConn1 -- Three-Phase V-I Measurement2/RConn2

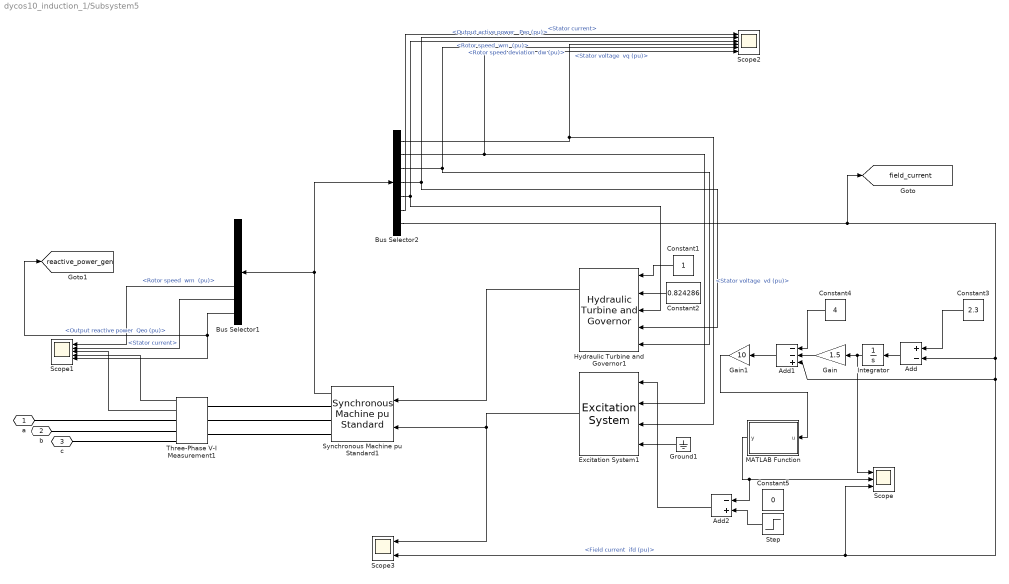
== system dycos10_induction_1/Subsystem5 ==
  Add : Sum  Inputs=+-
  Add1 : Sum  Inputs=--+
  Add2 : Sum  Inputs=-+
  Bus Selector1 : BusSelector  OutputSignals="dq0 components.Stator voltage  vd (pu),dq0 components.Stator voltage  vq (pu),Mechanical.Rotor speed deviation  dw (pu),Output active power   Peo (pu),Mechanical.Rotor speed  wm  (pu),Stator current,Output reactive power  Qeo (pu)"
  Bus Selector2 : BusSelector  OutputSignals="dq0 components.Stator voltage  vd (pu),dq0 components.Stator voltage  vq (pu),Mechanical.Rotor speed deviation  dw (pu),Output active power   Peo (pu),Mechanical.Rotor speed  wm  (pu),Stator current,dq0 components.Field current  ifd (pu)"
  Constant1 : Constant
  Constant2 : Constant  Value=0.824286
  Constant3 : Constant  Value=2.3
  Constant4 : Constant  Value=4
  Constant5 : Constant  Value=0
  Excitation System1 : powerlib/Machines/Excitation System  tr=20e-3  reg=[ 300, 0.001 ]  exc=[ 1, 0 ]  tgr=[ 0, 0 ]  damp=[ 0.001, 0.1 ]  sat=[ 0, 0 ]  lim=[ -11.5, 11.5, 0 ]  v0=[1,1.75396]
  Gain : Gain  Gain=1.5
  Gain1 : Gain  Gain=10
  Ground1 : Ground
  Hydraulic Turbine and Governor1 : powerlib/Machines/Hydraulic Turbine and Governor  sm="[ 10/3  0.07 ]"  gate="[  0.01  0.97518  -0.1  0.1 ]"  reg="[  0.05  1.163  0.105  0  0.01  ]"  hyd="[  0  2.67  ]"  dref=0  po=0.829511
  Integrator : Integrator  LimitOutput=on  UpperSaturationLimit=0  LowerSaturationLimit=-40
  MATLAB Function : MATLAB Function  TreatAsAtomicUnit=on
  Scope : Scope  NumInputPorts=3
  Scope1 : Scope  NumInputPorts=5
  Scope2 : Scope  NumInputPorts=6
  Scope3 : Scope  NumInputPorts=2
  Step : Step  Time=0  Before=1  SampleTime=0
  Synchronous Machine pu Standard1 : powerlib/Machines/Synchronous Machine pu Standard  PresetModel=No  MechanicalLoad=Mechanical power Pm  ShowDetailedParameters=on  RotorType=Salient-pole  Units=per unit standard parameters  MeasurementBus=off  NominalParameters=[1400e+06 24000 60]  Reactances1=[ 1.81, 0.3, 0.23, 1.76, 0.65, 0.25, 0.15 ]  Reactances2=[2.07 0.28 0.215 1.99 0.215 0.155]  dAxisTimeConstants=Open-circuit  qAxisTimeConstants=Open-circuit  TimeConstants1="[ 4.1  0.033  0.062  ]"  TimeConstants2=[ 8.0, 0.03, 1.0, 0.07 ]  TimeConstants3="[  4.49  0.0681  0.0513  ]"  TimeConstants4=[ 8.0, 0.03, 0.3371, 0.0295 ]  TimeConstants5=[ 1.01, 0.053, 0.1 ]  TimeConstants6=[ 1.3201, 0.023, 1.0, 0.07 ]  TimeConstants7=[4.1 0.033 0.062]  TimeConstants8=[ 1.3201, 0.0231, 0.3371, 0.0295 ]  StatorResistance=0.0046  Mechanical=[2.33 0 2]  PolePairs=20  InitialConditions=[0 24.3076 1.06584 1.06584 1.06584 51.9333 -68.0667 171.933 1.75396]  SetSaturation=off  Saturation=[0.6404,0.7127,0.8441,0.9214,0.9956,1.082,1.19,1.316,1.457;0.7,0.7698,0.8872,0.9466,0.9969,1.046,1.1,1.151,1.201]  LoadFlowParameters=[1 1154000000 0 0 0]  TsPowergui=0  TsBlock=-1  IterativeModel=Trapezoidal non iterative  IterativeDiscreteModel=Trapezoidal non iterative  BusType=PV  Pref=1154000000  Qref=0  Qmin=-Inf  Qmax=Inf  PLF=0  QLF=0
  Three-Phase V-I Measurement1 : powerlib/Measurements/Three-Phase V-I Measurement  VoltageMeasurement=phase-to-ground  SetLabelV=off  LabelV=Vabc  Vpu=on  VpuLL=off  CurrentMeasurement=yes  SetLabelI=off  LabelI=Iabc  Ipu=on  Pbase=1400e6  Vbase=24e3  OutputType=Magnitude  PhasorSimulation=on  PSBequivalent=0
  a : PMIOPort  Side=Right
  b : PMIOPort  Port=2  Side=Right
  c : PMIOPort  Port=3  Side=Right
  tag scope: field_current=global, reactive_power_gen=global
  wires:
  Three-Phase V-I Measurement1/1 -> Scope1/4
  Bus Selector2/1 -> Excitation System1/3, Scope2/4  "<Stator voltage  vd (pu)>"
  Three-Phase V-I Measurement1/2 -> Scope1/3
  Bus Selector2/6 -> Scope2/1  "<Stator current>"
  Hydraulic Turbine and Governor1/1 -> Synchronous Machine pu Standard1/1
  Bus Selector2/3 -> Hydraulic Turbine and Governor1/5, Scope2/5  "<Rotor speed deviation  dw (pu)>"
  Bus Selector2/4 -> Hydraulic Turbine and Governor1/4, Scope2/2  "<Output active power   Peo (pu)>"
  Constant1/1 -> Hydraulic Turbine and Governor1/1
  Bus Selector2/5 -> Hydraulic Turbine and Governor1/3, Scope2/3  "<Rotor speed  wm  (pu)>"
  Excitation System1/1 -> Scope3/1, Synchronous Machine pu Standard1/2
  Constant2/1 -> Hydraulic Turbine and Governor1/2
  Bus Selector2/2 -> Excitation System1/2, Scope2/6  "<Stator voltage  vq (pu)>"
  Bus Selector1/5 -> Scope1/1  "<Rotor speed  wm  (pu)>"
  Synchronous Machine pu Standard1/1 -> Bus Selector2/1, Bus Selector1/1
  Bus Selector1/6 -> Scope1/2  "<Stator current>"
  Ground1/1 -> Excitation System1/4
  Gain1/1 -> MATLAB Function/1(u)
  Constant4/1 -> Add1/1
  Add1/1 -> Gain1/1
  Gain/1 -> Add1/2
  Integrator/1 -> Scope/1, Gain/1
  Constant3/1 -> Add/1
  Add/1 -> Integrator/1
  Step/1 -> Add2/2
  Add2/1 -> Excitation System1/1
  MATLAB Function/1(y) -> Add2/1, Scope/2
  Bus Selector2/7 -> [field_current], Add/2, Add1/3, Scope/3, Scope3/2  "<Field current  ifd (pu)>"
  Bus Selector1/7 -> [reactive_power_gen], Scope1/5  "<Output reactive power  Qeo (pu)>"
  connections:
  Three-Phase V-I Measurement1/RConn1 -- a/RConn1
  Three-Phase V-I Measurement1/LConn2 -- Synchronous Machine pu Standard1/RConn2
  Three-Phase V-I Measurement1/RConn2 -- b/RConn1
  Three-Phase V-I Measurement1/LConn1 -- Synchronous Machine pu Standard1/RConn1
  Three-Phase V-I Measurement1/LConn3 -- Synchronous Machine pu Standard1/RConn3
  Three-Phase V-I Measurement1/RConn3 -- c/RConn1

== matlab function Subsystem5/MATLAB Function ==
  data: u input double; y output double
function y = fcn(u)
if u>0 
    y = u;
else 
    y=0;
end
